simulink model "systemSim"  (R2014a)
settings: Solver=ode45  StartTime=0.0  StopTime=500  MaxStep=.01  RelTol=1e-3
libraries: simulink x5
settings Model: Creator=a01225128  LastModifiedBy=a01225128

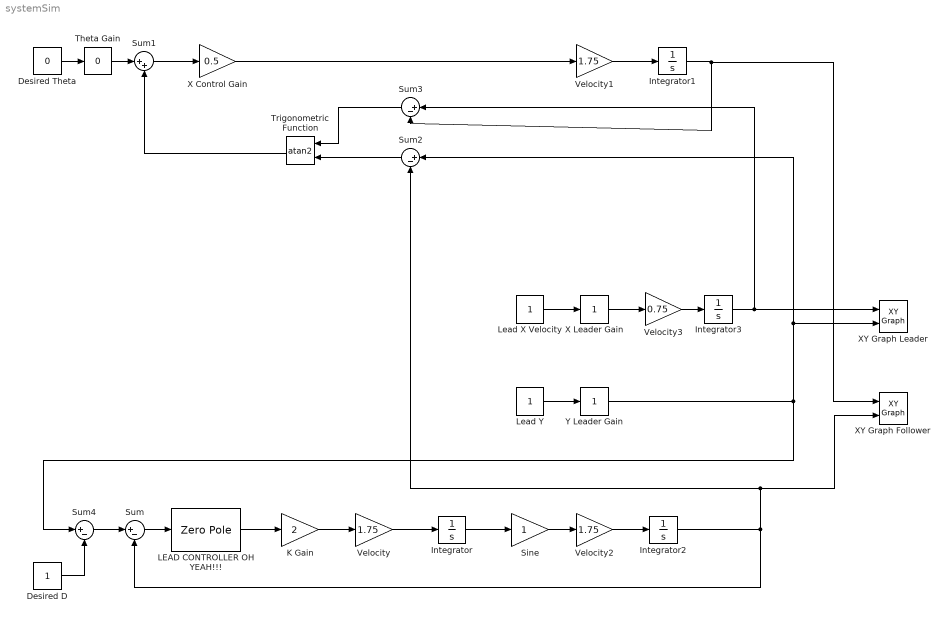
== system systemSim ==
  Desired D : Constant
  "Desired Theta " : Constant  Value=0
  Integrator{,1..3} (4 alike) : Integrator
  "K Gain " : Gain  Gain=2
  LEAD CONTROLLER OH YEAH!!! : ZeroPole  Zeros=[-0.6369]  Poles=[-4.8081]  Gain=[0.364]
  "Lead X Velocity " : Constant
  "Lead Y " : Constant
  "Sine " : Gain
  Sum{,2..4} (4 alike) : Sum  Inputs=|+-
  Sum1 : Sum  Inputs=|++
  "Theta Gain " : simulink/Math Operations/Slider Gain  low=-5  gain=0  high=5
  Trigonometric Function : Trigonometry  Operator=atan2
  Velocity : Gain  Gain=1.75
  Velocity1 : Gain  Gain=1.75
  Velocity2 : Gain  Gain=1.75
  Velocity3 : Gain  Gain=0.75
  "X Control Gain " : Gain  Gain=0.5
  "X Leader Gain " : simulink/Math Operations/Slider Gain  low=-5  gain=1  high=5
  "XY Graph Follower " : simulink/Sinks/XY Graph  xmin=-5  xmax=50  ymin=-10  ymax=10  st=-1
  XY Graph Leader : simulink/Sinks/XY Graph  xmin=-5  xmax=50  ymin=-10  ymax=10  st=-1
  "Y Leader Gain " : simulink/Math Operations/Slider Gain  low=-5  gain=1  high=10
  wires:
  Integrator/1 -> "Sine "/1
  Velocity/1 -> Integrator/1
  Integrator1/1 -> "XY Graph Follower "/1, Sum3/2
  Integrator2/1 -> Sum/2, "XY Graph Follower "/2, Sum2/2
  "Sine "/1 -> Velocity2/1
  Velocity2/1 -> Integrator2/1
  Velocity1/1 -> Integrator1/1
  Sum/1 -> LEAD CONTROLLER OH YEAH!!!/1
  "K Gain "/1 -> Velocity/1
  LEAD CONTROLLER OH YEAH!!!/1 -> "K Gain "/1
  "Theta Gain "/1 -> Sum1/1
  "Desired Theta "/1 -> "Theta Gain "/1
  Sum1/1 -> "X Control Gain "/1
  "X Control Gain "/1 -> Velocity1/1
  "Lead Y "/1 -> "Y Leader Gain "/1
  "Lead X Velocity "/1 -> "X Leader Gain "/1
  Velocity3/1 -> Integrator3/1
  Integrator3/1 -> XY Graph Leader/1, Sum3/1
  Sum3/1 -> Trigonometric Function/1
  Sum2/1 -> Trigonometric Function/2
  Trigonometric Function/1 -> Sum1/2
  "Y Leader Gain "/1 -> Sum4/1, XY Graph Leader/2, Sum2/1
  Desired D/1 -> Sum4/2
  Sum4/1 -> Sum/1
  "X Leader Gain "/1 -> Velocity3/1
